simulink model "dbm_2020b_em_test01"  (R2021b)
settings: Solver=VariableStepAuto  StartTime=0.0  StopTime=20  MaxStep=0.02  MinStep=0.002  RelTol=1e-3
libraries: autolibshared x1
settings Model: Creator=felix  LastModifiedBy=emilo
settings SolverCC: InitialStep=0.01  AlgebraicLoopSolver=TrustRegion

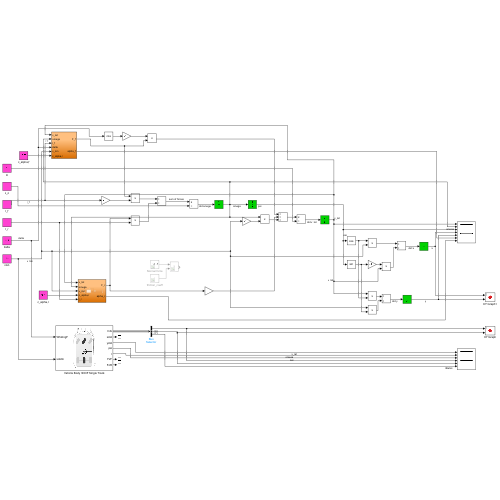
[thumbnail: Simulink's stored preview of the top-level diagram]
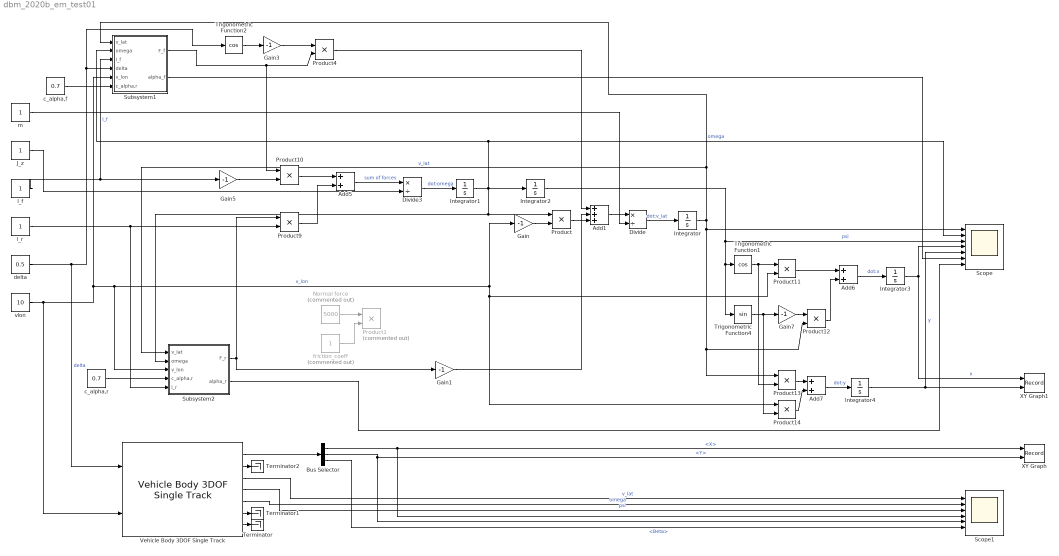
== system dbm_2020b_em_test01 ==
  Add1 : Sum  Inputs=+++
  Add5 : Sum
  Add6 : Sum
  Add7 : Sum
  Bus Selector : BusSelector  OutputSignals=InertFrm.Cg.Disp.X,InertFrm.Cg.Disp.Y,BdyFrm.Cg.Ang.Beta
  Divide : Product  Inputs=*/
  Divide3 : Product  Inputs=*/
  Gain{,1,3,5,7} (5 alike) : Gain  Gain=-1
  Integrator{,1..4} (5 alike) : Integrator
  J_z : Constant
  Normal force : Constant  Commented=on  Value=5000
  Product{,4,9..14} (8 alike) : Product
  Product1 : Product  Commented=on
  Scope : Scope  NumInputPorts=7
  Scope1 : Scope  NumInputPorts=6
  Subsystem1 : Subsystem
  Subsystem2 : Subsystem
  Terminator : Terminator
  Terminator1 : Terminator
  Terminator2 : Terminator
  Trigonometric Function1 : Trigonometry  Operator=cos
  Trigonometric Function2 : Trigonometry  Operator=cos
  Trigonometric Function4 : Trigonometry
  Vehicle Body 3DOF Single Track : autolibshared/Vehicle Body 3DOF Single Track  trackMode=Single (bicycle)  inputMode=External longitudinal velocity  frontSteerMode=on  rearSteerMode=off  windMode=off  muMode=off  extFMode=off  extMMode=off  htchFMode=off  htchMMode=off  extXo=off  extpsio=off  extxdoto=off  extro=off  extYo=off  extTamb=off  extydoto=off  aMode=2  NF=1  NR=1  m=1  a=1  b=1  h=0  dh=1  hh=0.2  X_o=0  xdot_o=0  CalphaMode=off  sigmaMode=off  d=0  hl=0  w=[1.4,1.4]  Cy_f=0.7  Cy_r=0.7  sigma_f=.1  sigma_r=.1  alpha_f_brk=[-.1 .1]  Cy_f_data=[-9e3 9e3]  alpha_r_brk=[-.1 .1]  Cy_r_data=[-9e3 9e3]  Y_o=0  ydot_o=0  Izz=1  psi_o=0  r_o=0  Af=0  Cd=0  Cl=0  Cpm=0  beta_w=[0:0.01:0.3]  Cs=[0:0.03:0.9]*0  Cym=[0:0.01:0.3]*0  Pabs=101325  Tair=273  g=9.81  mu=1  xdot_tol=.01  Fznom=9.81  Fxtire_sat=7e4  Fytire_sat=7e4  longOff=0  latOff=0  vertOff=0  wrapAng=off
      settings: SourceProductBaseCode=PW,DR,MT,UV,VE
  XY Graph : Record  FileSettingsInternal="{\"entries\":[{\"content\":{\"excelSettings\":{\"content\":{},\"type\":\"Streamout.ExcelSettings\"}},\"type\":\"Streamout.FileSettingStorage\",\"uuid\":\"75c249bf-30f8-4b23-abf8-bdf55cae673c\"}],\"packageUris\":[\"http://schema.mathworks.com/mf0/streamout_blocks/R2020a\"],\"version\":\"1.0\"}"  Layout=[1 1]  SignalsInternal="{\"entries\":[{\"content\":{\"signals\":[{\"content\":{\"blockPath\":[\"dbm_2020b_em_test01/XY Graph\"],\"channel\":[],\"dimensions\":[1],\"domain\":\"dbm_2020b_em_test01/XY Graph\",\"lineColor\":\"#a2142f\",\"plots\":[1],\"port\":1,\"sid\":[\"\"],\"signalID\":1597,\"signalName\":\"<X>\"},\"type\":\"RecordBlkView.Signal\",\"uuid\":\"13f576fb-e383-42ca-bcda-1c6612951e20\"},{\"content\":{\"blockPath\":[\"dbm_2020b_em_test01/XY Graph\"],\"channel\":[],\"dimensions\":[1],\"domain\":\"dbm_2020b_em_test01/XY Graph\",\"lineColor\":\"#139fff\",\"plots\":[1],\"port\":2,\"sid\":[\"\"],\"signalID\":1601,\"signalName\":\"<Y>\"},\"type\":\"RecordBlkView.Signal\",\"uuid\":\"a2425947-ff50-4901-b9b3-7f5b71d71a0b\"}]},\"type\":\"RecordBlkView.InputSignals\",\"uuid\":\"b4778b0f-135f-461e-95ec-15bf9516e1f1\"}],\"packageUris\":[\"http://schema.mathworks.com/mf0/streamout_blocks/R2020a\"],\"version\":\"1.0\"}"  VisualizationBindings="{\"xyplotplugin\":{\"info\":[{\"series\":[{\"bindingParametersList\":[{\"parameter\":\"X-Axis\",\"signalID\":1597,\"signalName\":\"<X>\"},{\"parameter\":\"Y-Axis\",\"signalID\":1601,\"signalName\":\"<Y>\"}],\"seriesID\":5838}],\"subplotID\":1}]}}"  CompatibilityTag=XY
  XY Graph1 : Record  FileSettingsInternal="{\"entries\":[{\"content\":{\"excelSettings\":{\"content\":{},\"type\":\"Streamout.ExcelSettings\"}},\"type\":\"Streamout.FileSettingStorage\",\"uuid\":\"0ccddee9-9aa5-42e1-954b-eb6b0415fe70\"}],\"packageUris\":[\"http://schema.mathworks.com/mf0/streamout_blocks/R2020a\"],\"version\":\"1.0\"}"  Layout=[1 1]  SignalsInternal="{\"entries\":[{\"content\":{\"signals\":[{\"content\":{\"blockPath\":[\"dbm_2020b_em_test01/XY Graph1\"],\"channel\":[],\"dimensions\":[1],\"domain\":\"dbm_2020b_em_test01/XY Graph1\",\"lineColor\":\"#a2142f\",\"plots\":[1],\"port\":1,\"sid\":[\"\"],\"signalID\":1605,\"signalName\":\"x\"},\"type\":\"RecordBlkView.Signal\",\"uuid\":\"2d517a74-843d-4e73-a2d5-137630aeccfb\"},{\"content\":{\"blockPath\":[\"dbm_2020b_em_test01/XY Graph1\"],\"channel\":[],\"dimensions\":[1],\"domain\":\"dbm_2020b_em_test01/XY Graph1\",\"lineColor\":\"#139fff\",\"plots\":[1],\"port\":2,\"sid\":[\"\"],\"signalID\":1609,\"signalName\":\"y\"},\"type\":\"RecordBlkView.Signal\",\"uuid\":\"9844b495-5393-4de3-944a-cb2ac91273bb\"}]},\"type\":\"RecordBlkView.InputSignals\",\"uuid\":\"b4ea2bd1-452d-4665-8b81-b915636b8195\"}],\"packageUris\":[\"http://schema.mathworks.com/mf0/streamout_blocks/R2020a\"],\"version\":\"1.0\"}"  VisualizationBindings="{\"xyplotplugin\":{\"info\":[{\"series\":[{\"bindingParametersList\":[{\"parameter\":\"X-Axis\",\"signalID\":1605,\"signalName\":\"x\"},{\"parameter\":\"Y-Axis\",\"signalID\":1609,\"signalName\":\"y\"}],\"seriesID\":20463}],\"subplotID\":1}]}}"  CompatibilityTag=XY
  c_alpha,f : Constant  Value=0.7
  c_alpha,r : Constant  Value=0.7
  delta : Constant  Value=0.5
  friction_coeff : Constant  Commented=on
  l_f : Constant
  l_r : Constant
  m : Constant
  vlon : Constant  Value=10
  wires:
  m/1 -> Divide/2
  Divide/1 -> Integrator/1  "dot:v_lat"
  Integrator/1 -> Product13/1, Product12/2, Scope/1, Subsystem1/1(v_lat), Subsystem2/1(v_lat)  "v_lat"
  Integrator1/1 -> Scope/2, Subsystem1/2(omega), Integrator2/1, Product/1, Subsystem2/2(omega)  "omega"
  vlon/1 -> Vehicle Body 3DOF Single Track/2, Subsystem2/3(v_lon), Product11/2, Product14/1, Gain/1, Subsystem1/5(v_lon)  "v_lon"
  Gain/1 -> Product/2
  l_r/1 -> Subsystem2/5(l_r), Product9/2
  Product/1 -> Add1/3
  delta/1 -> Vehicle Body 3DOF Single Track/1, Trigonometric Function2/1, Subsystem1/4(delta)  "delta"
  Trigonometric Function2/1 -> Gain3/1
  Gain3/1 -> Product4/1
  l_f/1 -> Gain5/1, Subsystem1/3(l_f)  "l_f"
  Add1/1 -> Divide/1
  J_z/1 -> Divide3/2
  Gain5/1 -> Product10/2
  Product10/1 -> Add5/1
  Product9/1 -> Add5/2
  Add5/1 -> Divide3/1  "sum of forces"
  Divide3/1 -> Integrator1/1  "dot:omega"
  Integrator2/1 -> Trigonometric Function4/1, Trigonometric Function1/1, Scope/3  "psi"
  Integrator3/1 -> XY Graph1/1, Scope/4  "x"
  Trigonometric Function1/1 -> Product11/1, Product13/2
  Product11/1 -> Add6/1
  Trigonometric Function4/1 -> Product14/2, Gain7/1
  Product12/1 -> Add6/2
  Add6/1 -> Integrator3/1  "dot:x"
  Integrator4/1 -> XY Graph1/2, Scope/5  "y"
  Product13/1 -> Add7/1
  Add7/1 -> Integrator4/1  "dot:y"
  Product14/1 -> Add7/2
  Gain7/1 -> Product12/1
  Product4/1 -> Add1/1
  Subsystem2/1(F_r) -> Gain1/1, Product9/1
  c_alpha,r/1 -> Subsystem2/4(c_alpha,r)
  Subsystem1/1(F_f) -> Product4/2, Product10/1
  c_alpha,f/1 -> Subsystem1/6(c_alpha,r)
  Vehicle Body 3DOF Single Track/2 -> Terminator2/1
  Vehicle Body 3DOF Single Track/3 -> Scope1/1  "v_lat"
  Vehicle Body 3DOF Single Track/5 -> Scope1/2  "omega"
  Vehicle Body 3DOF Single Track/4 -> Scope1/3  "psi"
  Vehicle Body 3DOF Single Track/7 -> Terminator/1
  Vehicle Body 3DOF Single Track/6 -> Terminator1/1
  Vehicle Body 3DOF Single Track/1 -> Bus Selector/1
  Bus Selector/1 -> XY Graph/1, Scope1/4  "<X>"
  Bus Selector/2 -> Scope1/5, XY Graph/2  "<Y>"
  friction_coeff/1 -> Product1/2
  Normal force/1 -> Product1/1
  Subsystem1/2(alpha_f) -> Scope/6
  Subsystem2/2(alpha_r) -> Scope/7
  Bus Selector/3 -> Scope1/6  "<Beta>"
  Gain1/1 -> Add1/2

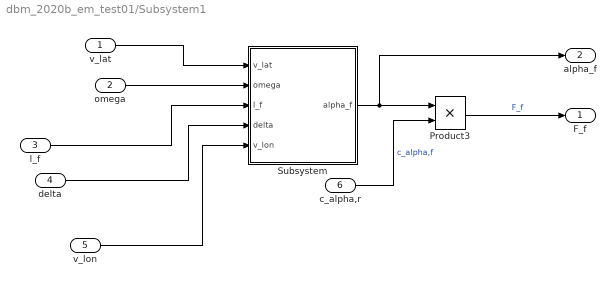
== system dbm_2020b_em_test01/Subsystem1 ==
  v_lat : Inport
  omega : Inport  Port=2
  l_f : Inport  Port=3
  delta : Inport  Port=4
  v_lon : Inport  Port=5
  c_alpha,r : Inport  Port=6
  Product3 : Product
  Subsystem : Subsystem
  F_f : Outport
  alpha_f : Outport  Port=2
  wires:
  Subsystem/1(alpha_f) -> alpha_f/1, Product3/1
  v_lat/1 -> Subsystem/1(v_lat)
  Product3/1 -> F_f/1  "F_f"
  v_lon/1 -> Subsystem/5(v_lon)
  c_alpha,r/1 -> Product3/2  "c_alpha,f"
  omega/1 -> Subsystem/2(omega)
  l_f/1 -> Subsystem/3(l_f)
  delta/1 -> Subsystem/4(delta)

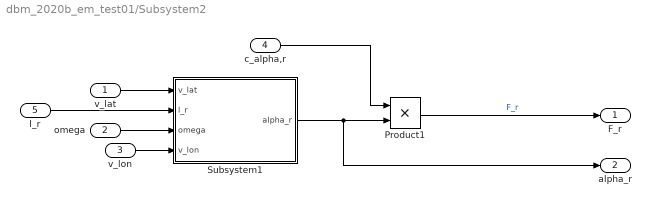
== system dbm_2020b_em_test01/Subsystem2 ==
  v_lat : Inport
  omega : Inport  Port=2
  v_lon : Inport  Port=3
  c_alpha,r : Inport  Port=4
  l_r : Inport  Port=5
  Product1 : Product
  Subsystem1 : Subsystem
  F_r : Outport
  alpha_r : Outport  Port=2
  wires:
  v_lat/1 -> Subsystem1/1(v_lat)
  c_alpha,r/1 -> Product1/1
  Subsystem1/1(alpha_r) -> alpha_r/1, Product1/2
  l_r/1 -> Subsystem1/2(l_r)
  omega/1 -> Subsystem1/3(omega)
  Product1/1 -> F_r/1  "F_r"
  v_lon/1 -> Subsystem1/4(v_lon)

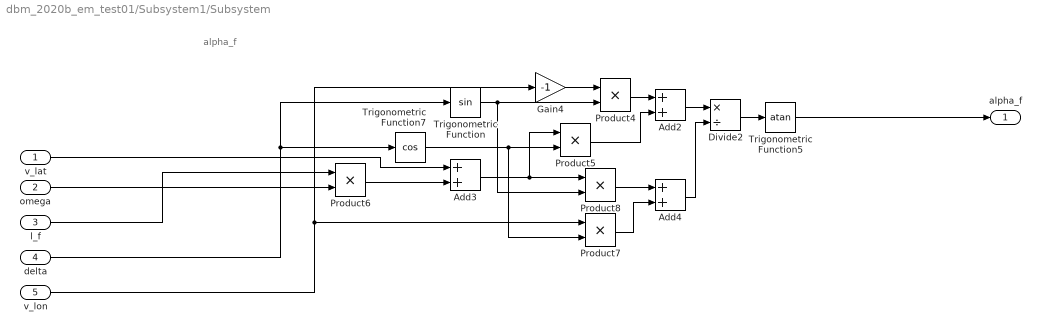
== system dbm_2020b_em_test01/Subsystem1/Subsystem ==
  note: alpha_f
  v_lat : Inport
  omega : Inport  Port=2
  l_f : Inport  Port=3
  delta : Inport  Port=4
  v_lon : Inport  Port=5
  Add2 : Sum
  Add3 : Sum
  Add4 : Sum
  Divide2 : Product  Inputs=*/
  Gain4 : Gain  Gain=-1
  Product{4..8} (5 alike) : Product
  Trigonometric Function : Trigonometry
  Trigonometric Function5 : Trigonometry  Operator=atan
  Trigonometric Function7 : Trigonometry  Operator=cos
  alpha_f : Outport
  wires:
  v_lon/1 -> Product7/1, Gain4/1
  Add2/1 -> Divide2/1
  Divide2/1 -> Trigonometric Function5/1
  Add4/1 -> Divide2/2
  Product5/1 -> Add2/2
  Trigonometric Function/1 -> Product8/2, Product4/2
  Product4/1 -> Add2/1
  Gain4/1 -> Product4/1
  Product6/1 -> Add3/2
  Add3/1 -> Product8/1, Product5/1
  delta/1 -> Trigonometric Function7/1, Trigonometric Function/1
  Product7/1 -> Add4/2
  v_lat/1 -> Add3/1
  Trigonometric Function7/1 -> Product7/2, Product5/2
  Product8/1 -> Add4/1
  l_f/1 -> Product6/1
  Trigonometric Function5/1 -> alpha_f/1
  omega/1 -> Product6/2

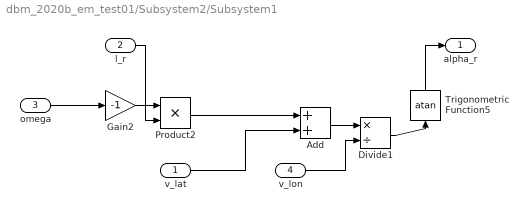
== system dbm_2020b_em_test01/Subsystem2/Subsystem1 ==
  v_lat : Inport
  l_r : Inport  Port=2
  omega : Inport  Port=3
  v_lon : Inport  Port=4
  Add : Sum
  Divide1 : Product  Inputs=*/
  Gain2 : Gain  Gain=-1
  Product2 : Product
  Trigonometric Function5 : Trigonometry  Operator=atan
  alpha_r : Outport
  wires:
  Divide1/1 -> Trigonometric Function5/1
  Add/1 -> Divide1/1
  l_r/1 -> Product2/2
  omega/1 -> Gain2/1
  Gain2/1 -> Product2/1
  v_lon/1 -> Divide1/2
  Product2/1 -> Add/1
  v_lat/1 -> Add/2
  Trigonometric Function5/1 -> alpha_r/1
